simulink model "Haerkegard_ActuatorDynamics"  (R2020b)
settings: Solver=VariableStepAuto  StartTime=0.0  StopTime=4  RelTol=1e-3
undefined symbols (not defined in the file): B, tfpred
libraries: qcatlib x1
settings Model: Creator=jeremie  LastModifiedBy=jeremie
settings DebuggingCC: ArithmeticOperatorsInVariantConditions=warning
settings SFSimCC: CustomCodeUndefinedFunction=UseInterfaceOnly

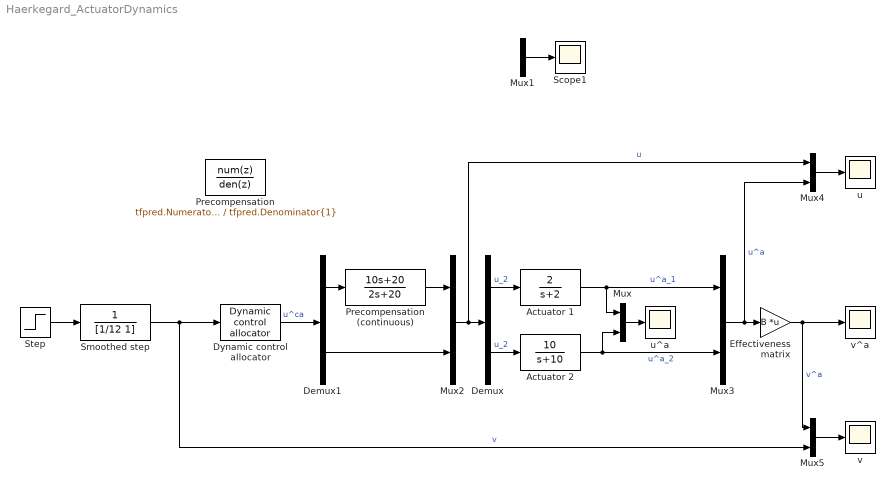
== system Haerkegard_ActuatorDynamics ==
  Actuator 1 : TransferFcn  Numerator=[2]  Denominator=[1 2]
  Actuator 2 : TransferFcn  Numerator=[10]  Denominator=[1 10]
  Demux : Demux  Outputs=2
  Demux1 : Demux  Outputs=2
  Dynamic control allocator : qcatlib/Dynamic control allocator  B=B  plim=[-1,1;-2,2]  rlim=[]  T=0.02  Wv=1  W1=diag([1,1])  W2=diag([12,0])  S=[0;0]
  Effectiveness matrix : Gain  Gain=B  Multiplication=Matrix(K*u)
  Mux{,1..5} (6 alike) : Mux  Inputs=2
  Precompensation : DiscreteTransferFcn  Numerator=tfpred.Numerator{1}  Denominator=tfpred.Denominator{1}  SampleTime=0.02
  Precompensation (continuous) : TransferFcn  Numerator=[10 20]  Denominator=[2 20]
  Scope1 : Scope
  Smoothed step : TransferFcn  Denominator=[1/12 1]
  Step : Step  Time=0.5  After=3  SampleTime=0
  u : Scope
  u^a : Scope
  v : Scope
  v^a : Scope
  wires:
  Actuator 1/1 -> Mux3/1, Mux/1  "u^a_1"
  Actuator 2/1 -> Mux/2, Mux3/2  "u^a_2"
  Mux/1 -> u^a/1
  Mux1/1 -> Scope1/1
  Demux/2 -> Actuator 2/1  "u_2"
  Demux/1 -> Actuator 1/1  "u_2"
  Mux2/1 -> Mux4/1, Demux/1  "u"
  Precompensation (continuous)/1 -> Mux2/1
  Demux1/2 -> Mux2/2
  Demux1/1 -> Precompensation (continuous)/1
  Dynamic control allocator/1 -> Demux1/1  "u^ca"
  Mux3/1 -> Mux4/2, Effectiveness matrix/1  "u^a"
  Effectiveness matrix/1 -> Mux5/1, v^a/1  "v^a"
  Step/1 -> Smoothed step/1
  Mux4/1 -> u/1
  Smoothed step/1 -> Mux5/2, Dynamic control allocator/1  "v"
  Mux5/1 -> v/1
